simulink model "equivalent_circuit_charge"  (R2013a)
settings: Solver=ode45  StartTime=0.0  StopTime=100  RelTol=1e-3
libraries: fl_lib x48, nesl_utility x18, elec_lib x12
settings Model: Creator=shrey  LastModifiedBy=shrey

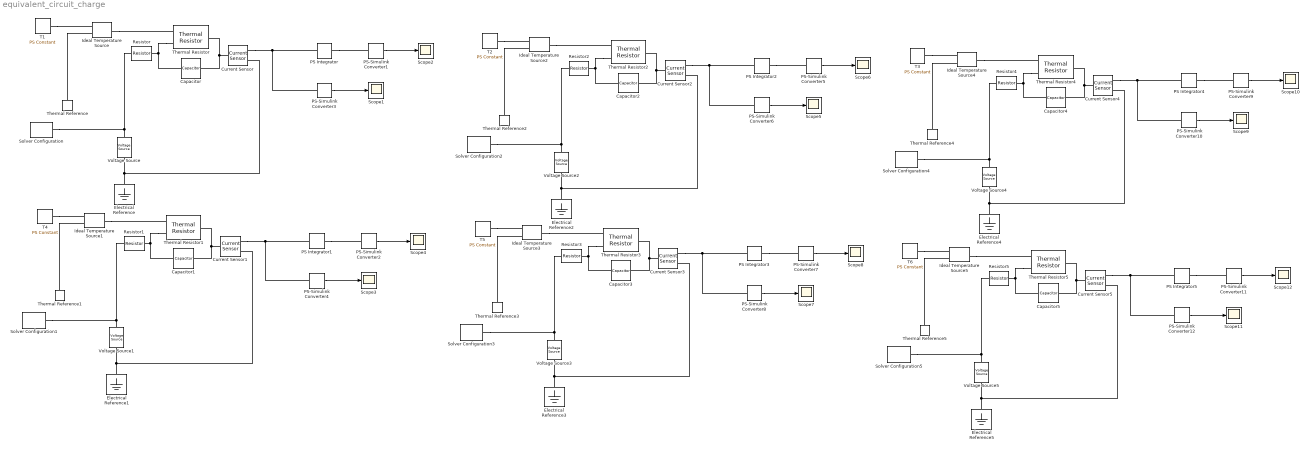
== system equivalent_circuit_charge ==
  Capacitor{,1..5} (6 alike) : fl_lib/Electrical/Electrical Elements/Capacitor  c=3600/4.2 F  v0=2.5 V  r=1e-6 Ohm  g=0 1/Ohm  i_Log=off  v_Log=off  vc_Log=off  LocalVarNames=|i|v|vc  LocalVarDescs=|i|v|Internal variable for voltage across capacitor term  LocalVarLogging=[0 0 0]
  Current Sensor{,1..5} (6 alike) : fl_lib/Electrical/Electrical Sensors/Current Sensor  i1_Log=off  v1_Log=off  LocalVarNames=|i1|v1  LocalVarDescs=|i1|v1  LocalVarLogging=[0 0]
  Electrical Reference{,1..5} (6 alike) : fl_lib/Electrical/Electrical Elements/Electrical Reference  i_Log=off  LocalVarNames=|i  LocalVarDescs=|i  LocalVarLogging=0
  Ideal Temperature Source{,1..5} (6 alike) : fl_lib/Thermal/Thermal Sources/Ideal Temperature Source  Q_Log=off  T_Log=off  LocalVarNames=|Q|T  LocalVarDescs=|Q|T  LocalVarLogging=[0 0]
  PS Integrator{,1..5} (6 alike) : fl_lib/Physical Signals/Linear Operators/PS Integrator  x0=0  x_Log=off  LocalVarNames=|x  LocalVarDescs=|x  LocalVarLogging=0
  PS-Simulink Converter{1..12} (12 alike) : nesl_utility/PS-Simulink Converter  PhysicalDomain=network_engine_domain  SubClassName=ps_output  LeftPortType=input  RightPortType=output  PseudoPeriodic=off  Frequencies=[]  Unit=1  AffineConversion=off
  Resistor{,1..5} (6 alike) : fl_lib/Electrical/Electrical Elements/Resistor  R=1 Ohm  i_Log=off  v_Log=off  LocalVarNames=|i|v  LocalVarDescs=|i|v  LocalVarLogging=[0 0]
  Scope{1..12} (12 alike) : Scope
      Scope1 settings: SaveName=Current
      Scope10 settings: SaveName=Charge4
      Scope11 settings: SaveName=Current5
      Scope12 settings: SaveName=Charge5
      Scope2 settings: SaveName=Charge
      Scope3 settings: SaveName=Current1
      Scope4 settings: SaveName=Charge1
      Scope5 settings: SaveName=Current2
      Scope6 settings: SaveName=Charge2
      Scope7 settings: SaveName=Current3
      Scope8 settings: SaveName=Charge3
      Scope9 settings: SaveName=Current4
  Solver Configuration{,1..5} (6 alike) : nesl_utility/Solver Configuration  PhysicalDomain=network_engine_domain  SubClassName=solver  LeftPortType=input  RightPortType=generic  Accelerate=off  Tones=[]  Harmonics=[]  SimulateNoise=off  Profile=off  UseLocalSampling=off  EnableSwitchedLinearOptims=on  FrequencyDomain=off  UseCCode=off  UseNewInitialization=off  DoDC=off  ResidualTolerance=1e-09  UseLocalSolver=on  LocalSolverChoice=NE_TRAPEZOIDAL_ADVANCER  LocalSolverSampleTime=0.001  DoFixedCost=on  MaxNonlinIter=3  MaxModeIter=2  LinearAlgebra=Sparse  DelaysMemoryBudget=1024
  T1 : fl_lib/Physical Signals/Sources/PS Constant  constant=253  LocalVarLogging=[]
  T2 : fl_lib/Physical Signals/Sources/PS Constant  constant=273  LocalVarLogging=[]
  T3 : fl_lib/Physical Signals/Sources/PS Constant  constant=293  LocalVarLogging=[]
  T4 : fl_lib/Physical Signals/Sources/PS Constant  constant=313  LocalVarLogging=[]
  T5 : fl_lib/Physical Signals/Sources/PS Constant  constant=333  LocalVarLogging=[]
  T6 : fl_lib/Physical Signals/Sources/PS Constant  constant=353  LocalVarLogging=[]
  Thermal Reference{,1..5} (6 alike) : fl_lib/Thermal/Thermal Elements/Thermal Reference  Q_Log=off  LocalVarNames=|Q  LocalVarDescs=|Q  LocalVarLogging=0
  Thermal Resistor{,1..5} (6 alike) : elec_lib/Passive Devices/Thermal Resistor  R0=7e-3 Ohm  T0=273 K  alpha=5e-5 1/K  tc=10 s  K_d=0.001 W/K  init_temp=25 C  current_Log=off  voltage_Log=off  power_Log=off  temperature_Log=off  heat_flow_Log=off  LocalVarNames=|current|voltage|power|temperature|heat_flow  LocalVarDescs=|Resistor current (A)|Voltage across resistor (V)|Power (W)|Thermistor temperature (K)|Heat flow (J/s)  LocalVarLogging=[0 0 0 0 0]
  Voltage Source : elec_lib/Sources/Voltage Source  dc_voltage=4.2 V  ac_voltage=0 V  ac_shift=0 deg  ac_frequency=60 Hz  noise_mode=1  PSD=0 V^2/Hz  sample_time=0.001 s  repeatability=1  auto_seed=802611725  user_seed=0  LocalVarLogging=[]
  Voltage Source1 : elec_lib/Sources/Voltage Source  dc_voltage=4.2 V  ac_voltage=0 V  ac_shift=0 deg  ac_frequency=60 Hz  noise_mode=1  PSD=0 V^2/Hz  sample_time=0.001 s  repeatability=1  auto_seed=1227669238  user_seed=0  LocalVarLogging=[]
  Voltage Source2 : elec_lib/Sources/Voltage Source  dc_voltage=4.2 V  ac_voltage=0 V  ac_shift=0 deg  ac_frequency=60 Hz  noise_mode=1  PSD=0 V^2/Hz  sample_time=0.001 s  repeatability=1  auto_seed=3252150220  user_seed=0  LocalVarLogging=[]
  Voltage Source3 : elec_lib/Sources/Voltage Source  dc_voltage=4.2 V  ac_voltage=0 V  ac_shift=0 deg  ac_frequency=60 Hz  noise_mode=1  PSD=0 V^2/Hz  sample_time=0.001 s  repeatability=1  auto_seed=3237241810  user_seed=0  LocalVarLogging=[]
  Voltage Source4 : elec_lib/Sources/Voltage Source  dc_voltage=4.2 V  ac_voltage=0 V  ac_shift=0 deg  ac_frequency=60 Hz  noise_mode=1  PSD=0 V^2/Hz  sample_time=0.001 s  repeatability=1  auto_seed=1634002471  user_seed=0  LocalVarLogging=[]
  Voltage Source5 : elec_lib/Sources/Voltage Source  dc_voltage=4.2 V  ac_voltage=0 V  ac_shift=0 deg  ac_frequency=60 Hz  noise_mode=1  PSD=0 V^2/Hz  sample_time=0.001 s  repeatability=1  auto_seed=2438775377  user_seed=0  LocalVarLogging=[]
  wires:
  PS-Simulink Converter3/1 -> Scope1/1
  PS-Simulink Converter1/1 -> Scope2/1
  PS-Simulink Converter4/1 -> Scope3/1
  PS-Simulink Converter2/1 -> Scope4/1
  PS-Simulink Converter6/1 -> Scope5/1
  PS-Simulink Converter5/1 -> Scope6/1
  PS-Simulink Converter8/1 -> Scope7/1
  PS-Simulink Converter7/1 -> Scope8/1
  PS-Simulink Converter10/1 -> Scope9/1
  PS-Simulink Converter9/1 -> Scope10/1
  PS-Simulink Converter12/1 -> Scope11/1
  PS-Simulink Converter11/1 -> Scope12/1
  connections:
  Thermal Resistor/LConn2 -- Capacitor/LConn1 -- Resistor/LConn1
  Thermal Resistor/RConn1 -- Current Sensor/LConn1 -- Capacitor/RConn1
  Solver Configuration/RConn1 -- Resistor/RConn1 -- Voltage Source/LConn1
  Voltage Source/RConn1 -- Current Sensor/RConn2 -- Electrical Reference/LConn1
  Thermal Reference/LConn1 -- Ideal Temperature Source/RConn2
  Ideal Temperature Source/LConn1 -- Thermal Resistor/LConn1
  T1/RConn1 -- Ideal Temperature Source/RConn1
  Current Sensor/RConn1 -- PS-Simulink Converter3/LConn1 -- PS Integrator/LConn1
  PS Integrator/RConn1 -- PS-Simulink Converter1/LConn1
  Thermal Resistor1/LConn2 -- Capacitor1/LConn1 -- Resistor1/LConn1
  Capacitor1/RConn1 -- Thermal Resistor1/RConn1 -- Current Sensor1/LConn1
  Solver Configuration1/RConn1 -- Resistor1/RConn1 -- Voltage Source1/LConn1
  Voltage Source1/RConn1 -- Current Sensor1/RConn2 -- Electrical Reference1/LConn1
  Current Sensor1/RConn1 -- PS-Simulink Converter4/LConn1 -- PS Integrator1/LConn1
  PS Integrator1/RConn1 -- PS-Simulink Converter2/LConn1
  T4/RConn1 -- Ideal Temperature Source1/RConn1
  Ideal Temperature Source1/LConn1 -- Thermal Resistor1/LConn1
  Thermal Reference1/LConn1 -- Ideal Temperature Source1/RConn2
  Thermal Resistor2/LConn2 -- Capacitor2/LConn1 -- Resistor2/LConn1
  Capacitor2/RConn1 -- Thermal Resistor2/RConn1 -- Current Sensor2/LConn1
  Solver Configuration2/RConn1 -- Resistor2/RConn1 -- Voltage Source2/LConn1
  Voltage Source2/RConn1 -- Current Sensor2/RConn2 -- Electrical Reference2/LConn1
  Current Sensor2/RConn1 -- PS-Simulink Converter6/LConn1 -- PS Integrator2/LConn1
  PS Integrator2/RConn1 -- PS-Simulink Converter5/LConn1
  Thermal Reference2/LConn1 -- Ideal Temperature Source2/RConn2
  Ideal Temperature Source2/LConn1 -- Thermal Resistor2/LConn1
  T2/RConn1 -- Ideal Temperature Source2/RConn1
  Thermal Resistor3/LConn2 -- Capacitor3/LConn1 -- Resistor3/LConn1
  Capacitor3/RConn1 -- Thermal Resistor3/RConn1 -- Current Sensor3/LConn1
  Solver Configuration3/RConn1 -- Resistor3/RConn1 -- Voltage Source3/LConn1
  Voltage Source3/RConn1 -- Current Sensor3/RConn2 -- Electrical Reference3/LConn1
  Current Sensor3/RConn1 -- PS-Simulink Converter8/LConn1 -- PS Integrator3/LConn1
  Thermal Reference3/LConn1 -- Ideal Temperature Source3/RConn2
  T5/RConn1 -- Ideal Temperature Source3/RConn1
  PS Integrator3/RConn1 -- PS-Simulink Converter7/LConn1
  Ideal Temperature Source3/LConn1 -- Thermal Resistor3/LConn1
  Thermal Resistor4/LConn2 -- Capacitor4/LConn1 -- Resistor4/LConn1
  Capacitor4/RConn1 -- Thermal Resistor4/RConn1 -- Current Sensor4/LConn1
  Solver Configuration4/RConn1 -- Resistor4/RConn1 -- Voltage Source4/LConn1
  Voltage Source4/RConn1 -- Current Sensor4/RConn2 -- Electrical Reference4/LConn1
  Current Sensor4/RConn1 -- PS-Simulink Converter10/LConn1 -- PS Integrator4/LConn1
  Thermal Reference4/LConn1 -- Ideal Temperature Source4/RConn2
  T3/RConn1 -- Ideal Temperature Source4/RConn1
  Ideal Temperature Source4/LConn1 -- Thermal Resistor4/LConn1
  PS Integrator4/RConn1 -- PS-Simulink Converter9/LConn1
  Thermal Resistor5/LConn2 -- Capacitor5/LConn1 -- Resistor5/LConn1
  Capacitor5/RConn1 -- Thermal Resistor5/RConn1 -- Current Sensor5/LConn1
  Solver Configuration5/RConn1 -- Resistor5/RConn1 -- Voltage Source5/LConn1
  Voltage Source5/RConn1 -- Current Sensor5/RConn2 -- Electrical Reference5/LConn1
  Current Sensor5/RConn1 -- PS-Simulink Converter12/LConn1 -- PS Integrator5/LConn1
  Thermal Reference5/LConn1 -- Ideal Temperature Source5/RConn2
  T6/RConn1 -- Ideal Temperature Source5/RConn1
  Ideal Temperature Source5/LConn1 -- Thermal Resistor5/LConn1
  PS Integrator5/RConn1 -- PS-Simulink Converter11/LConn1
